simulink model "Ida_FrameWork_Loop"  (R2023a)
settings: Solver=VariableStepAuto  StartTime=0.0  StopTime=inf  RelTol=1e-3
InitFcn:
  | run("Ida_Dynamic.mlx")
undefined symbols (not defined in the file): Cables, Design, init, kappa, n_time_sample, Path, sim_time
libraries: simulink x1
settings Model: PauseTimes=0.01  Creator=Saman  LastModifiedBy=Saman
settings DebuggingCC: UnderSpecifiedDimensionMsg=warning

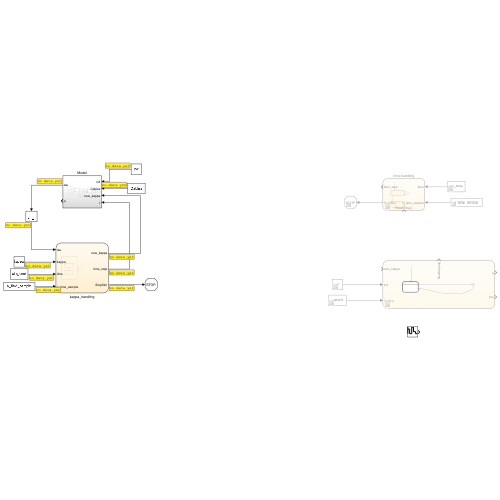
[thumbnail: Simulink's stored preview of the top-level diagram]
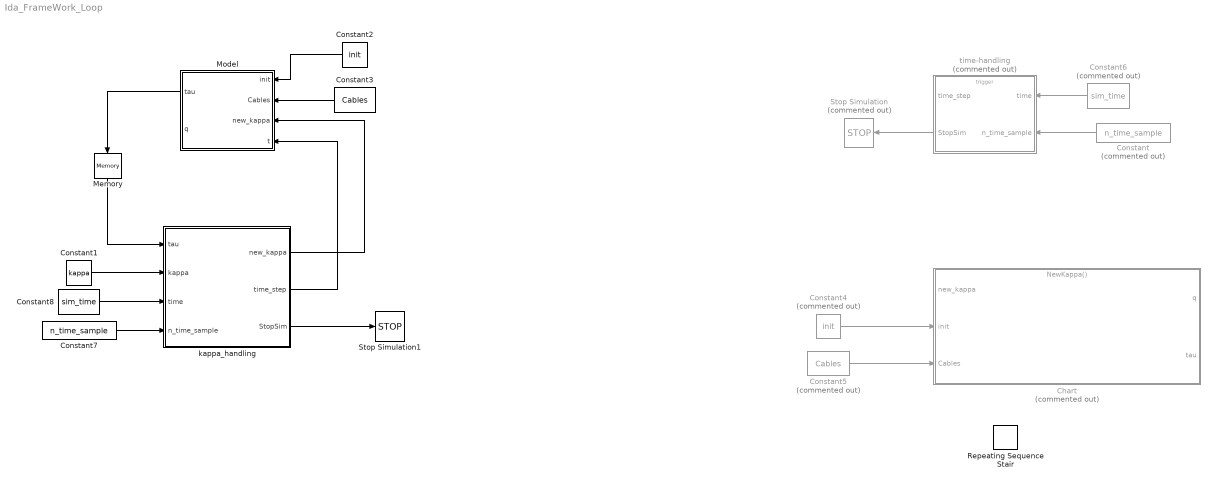
== system Ida_FrameWork_Loop ==
  Chart : Stateflow chart  Commented=on  TreatAsAtomicUnit=on
      settings: PortSchema="{\"entries\":[{\"content\":{\"sides\":[{\"content\":{\"connectorIds\":[\"In1\",\"In2\",\"In3\"]},\"type\":\"ConnectorPlacement.EquallySpacedRectSide\",\"uuid\":\"191c1550-6bd7-40a1-a407-faed922c01f5\"},{\"content\":{\"connectorIds\":[\"Out1\",\"Out2\"],\"side\":\"RIGHT\"},\"type\":\"ConnectorPlacement.EquallySpacedRectSide\",\"uuid\":\"ea9eb825-e49b-447b-9f77-f893937989a1\"},{\"content\":{\"connectorIds\":[\"Out3\"],\"side\":\"TOP\"},\"type\":\"ConnectorPlacement.EquallySpacedRectSide\",\"uuid\":\"63a28030-9dfb-4068-964b-2b00dab3f248\"}]},\"type\":\"ConnectorPlacement.EquallySpacedConnector\",\"uuid\":\"82f8fa03-3b4f-46da-8e57-1f2771fc7109\"}],\"packageUris\":[\"http://schema.mathworks.com/mf0/Connector/R2020b\"],\"version\":\"1.0\"}"
  Constant : Constant  Commented=on  Value=n_time_sample
  Constant1 : Constant  Value=kappa
  Constant2 : Constant  Value=init  OutDataTypeStr=Bus: slBus3
  Constant3 : Constant  Value=Cables  OutDataTypeStr=Bus: slBus1
  Constant4 : Constant  Commented=on  Value=init  OutDataTypeStr=Bus: slBus3
  Constant5 : Constant  Commented=on  Value=Cables  OutDataTypeStr=Bus: slBus1
  Constant6 : Constant  Commented=on  Value=sim_time
  Constant7 : Constant  Value=n_time_sample
  Constant8 : Constant  Value=sim_time
  Memory : Memory
  Model : Subsystem
  Repeating Sequence Stair : simulink/Sources/Repeating Sequence Stair  OutValues=sim_time  tsamp=-1  OutMin=[]  OutMax=[]  OutDataTypeStr=double  OutputDataTypeScalingMode=double  OutDataType=fixdt(0,8)  ConRadixGroup=Best Precision: Vector-wise  OutScaling=2^-12
  Stop Simulation : Stop  Commented=on
  Stop Simulation1 : Stop
  kappa_handling : Stateflow chart  TreatAsAtomicUnit=on
  time-handling : Stateflow chart  Commented=on  TreatAsAtomicUnit=on
  wires:
  Constant4/1 -> Chart/2(init)
  Constant5/1 -> Chart/3(Cables)
  Constant1/1 -> kappa_handling/2(kappa)
  Model/1(tau) -> Memory/1
  Constant3/1 -> Model/2(Cables)
  Constant2/1 -> Model/1(init)
  kappa_handling/1(new_kappa) -> Model/3(new_kappa)
  Memory/1 -> kappa_handling/1(tau)
  Constant6/1 -> time-handling/1(time)
  Constant/1 -> time-handling/2(n_time_sample)
  time-handling/2(StopSim) -> Stop Simulation/1
  kappa_handling/3(StopSim) -> Stop Simulation1/1
  Constant8/1 -> kappa_handling/3(time)
  Constant7/1 -> kappa_handling/4(n_time_sample)
  kappa_handling/2(time_step) -> Model/4(t)

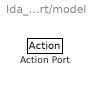
== system Ida_FrameWork_Loop/Chart/model ==
  Action Port : ActionPort
      settings: CopyFcn=Stateflow.SLINSF.SimulinkMan.removeBlockPreDeleteFcn  PreDeleteFcn=Stateflow.SLINSF.SimulinkMan.unsafePredeleteFcn

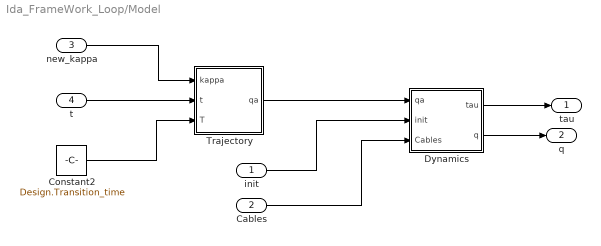
== system Ida_FrameWork_Loop/Model ==
  init : Inport
  Cables : Inport  Port=2
  new_kappa : Inport  Port=3
  t : Inport  Port=4
  Constant2 : Constant  Value=Design.Transition_time
  Dynamics : Subsystem
  Trajectory : Subsystem
  tau : Outport
  q : Outport  Port=2
  wires:
  new_kappa/1 -> Trajectory/1(kappa)
  Dynamics/1(tau) -> tau/1
  Dynamics/2(q) -> q/1
  t/1 -> Trajectory/2(t)
  init/1 -> Dynamics/2(init)
  Cables/1 -> Dynamics/3(Cables)
  Trajectory/1(qa) -> Dynamics/1(qa)
  Constant2/1 -> Trajectory/3(T)

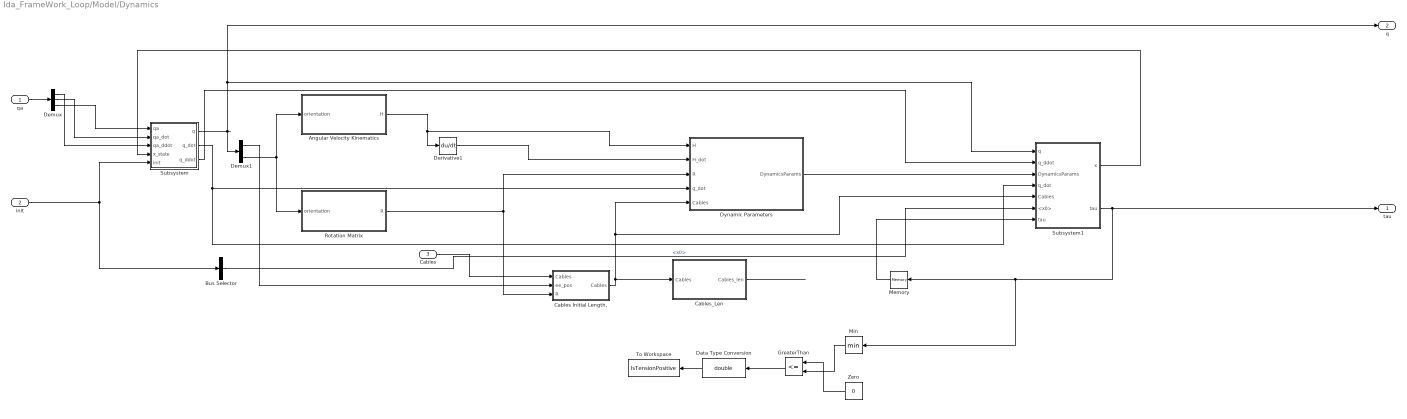
== system Ida_FrameWork_Loop/Model/Dynamics ==
  qa : Inport
  init : Inport  Port=2  OutDataTypeStr=Bus: slBus3
  Cables : Inport  Port=3  OutDataTypeStr=Bus: slBus1
  Angular Velocity Kinematics : MATLAB Function  TreatAsAtomicUnit=on
  Bus Selector : BusSelector  OutputSignals=x0
  Cables Initial Length, : MATLAB Function  TreatAsAtomicUnit=on
  Cables_Len : MATLAB Function  TreatAsAtomicUnit=on
  Data Type Conversion : DataTypeConversion  OutDataTypeStr=double  SaturateOnIntegerOverflow=off  RndMeth=Floor
  Demux : Demux  Outputs=3
  Demux1 : Demux  Outputs=2
  Derivative1 : Derivative
  Dynamic Parameters : MATLAB Function  TreatAsAtomicUnit=on
  GreaterThan : RelationalOperator  Operator=<=  OutDataTypeStr=boolean  RndMeth=Simplest  InputSameDT=off
  Memory : Memory
  Min : MinMax
  Rotation Matrix : MATLAB Function  TreatAsAtomicUnit=on
  Subsystem : Subsystem
  Subsystem1 : Subsystem
  To Workspace : ToWorkspace  VariableName=IsTensionPositive  SaveFormat=Timeseries  SampleTime=-1
  Zero : Constant  Value=0  OutDataTypeStr=Inherit: Inherit via back propagation
  tau : Outport
  q : Outport  Port=2
  wires:
  Cables/1 -> Cables Initial Length,/1("Cables ")
  Angular Velocity Kinematics/1(H) -> Dynamic Parameters/1(H), Derivative1/1
  Derivative1/1 -> Dynamic Parameters/2(H_dot)
  Rotation Matrix/1(R) -> Cables Initial Length,/3(R), Dynamic Parameters/3(R)
  qa/1 -> Demux/1
  init/1 -> Bus Selector/1, Subsystem/5(init)
  Subsystem/1(q) -> q/1, Subsystem1/1(q), Demux1/1
  Demux1/2 -> Rotation Matrix/1(orientation), Angular Velocity Kinematics/1(orientation)
  Demux1/1 -> Cables Initial Length,/2(ee_pos)
  Subsystem/2(q_dot) -> Subsystem1/4(q_dot), Dynamic Parameters/4(q_dot)
  Demux/3 -> Subsystem/1(qa)
  Demux/2 -> Subsystem/2(qa_dot)
  Demux/1 -> Subsystem/3(qa_ddot)
  GreaterThan/1 -> Data Type Conversion/1
  Zero/1 -> GreaterThan/1
  Min/1 -> GreaterThan/2
  Cables Initial Length,/1(Cables) -> Cables_Len/1(Cables), Subsystem1/5(Cables), Dynamic Parameters/5(Cables)
  Cables_Len/1(Cables_len) -> ?
  Data Type Conversion/1 -> To Workspace/1
  Subsystem1/2(tau) -> tau/1, Min/1, Memory/1
  Subsystem/3(q_ddot) -> Subsystem1/2(q_ddot)
  Dynamic Parameters/1(DynamicsParams) -> Subsystem1/3(DynamicsParams)
  Bus Selector/1 -> Subsystem1/6(<x0>)  "<x0>"
  Memory/1 -> Subsystem1/7("tau ")
  Subsystem1/1(x) -> Subsystem/4(x_state)

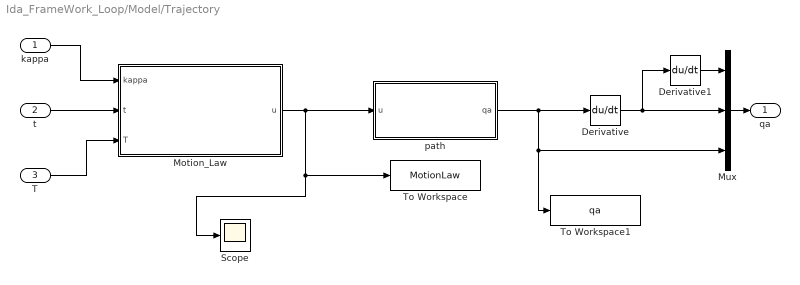
== system Ida_FrameWork_Loop/Model/Trajectory ==
  kappa : Inport
  t : Inport  Port=2
  T : Inport  Port=3
  Derivative : Derivative
  Derivative1 : Derivative
  Motion_Law : MATLAB Function  TreatAsAtomicUnit=on
  Mux : Mux  Inputs=3
  Scope : Scope
  To Workspace : ToWorkspace  VariableName=MotionLaw  SaveFormat=Timeseries  SampleTime=-1
  To Workspace1 : ToWorkspace  VariableName=qa  SaveFormat=Timeseries  SampleTime=-1
  path : MATLAB Function  TreatAsAtomicUnit=on
  qa : Outport
  wires:
  Derivative1/1 -> Mux/1
  Motion_Law/1(u) -> Scope/1, To Workspace/1, path/1(u)
  Derivative/1 -> Derivative1/1, Mux/2
  path/1(qa) -> Derivative/1, To Workspace1/1, Mux/3
  T/1 -> Motion_Law/3(T)
  t/1 -> Motion_Law/2(t)
  Mux/1 -> qa/1
  kappa/1 -> Motion_Law/1(kappa)

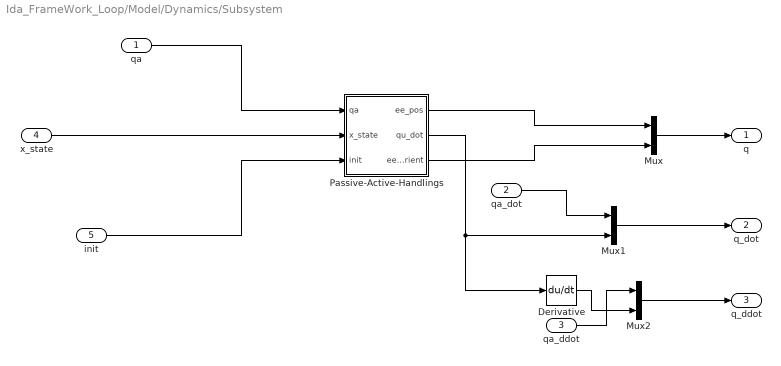
== system Ida_FrameWork_Loop/Model/Dynamics/Subsystem ==
  qa : Inport
  qa_dot : Inport  Port=2
  qa_ddot : Inport  Port=3
  x_state : Inport  Port=4
  init : Inport  Port=5
  Derivative : Derivative
  Mux : Mux  Inputs=2
  Mux1 : Mux  Inputs=2
  Mux2 : Mux  Inputs=2
  Passive-Active-Handlings : Stateflow chart  TreatAsAtomicUnit=on
  q : Outport
  q_dot : Outport  Port=2
  q_ddot : Outport  Port=3
  wires:
  qa/1 -> Passive-Active-Handlings/1(qa)
  Passive-Active-Handlings/3(ee_orient) -> Mux/2
  x_state/1 -> Passive-Active-Handlings/2(x_state)
  init/1 -> Passive-Active-Handlings/3(init)
  Passive-Active-Handlings/1(ee_pos) -> Mux/1
  Mux/1 -> q/1
  qa_dot/1 -> Mux1/1
  Passive-Active-Handlings/2(qu_dot) -> Derivative/1, Mux1/2
  Mux1/1 -> q_dot/1
  Mux2/1 -> q_ddot/1
  qa_ddot/1 -> Mux2/1
  Derivative/1 -> Mux2/2

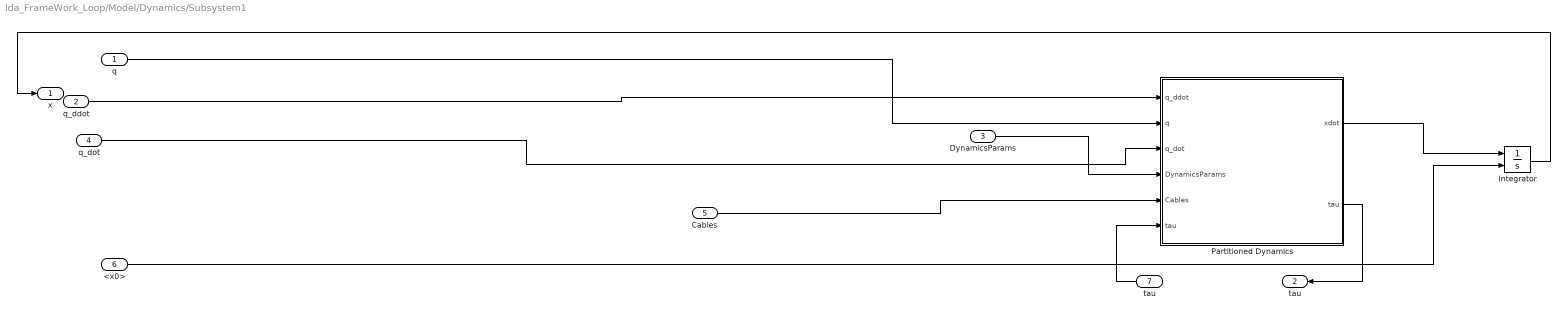
== system Ida_FrameWork_Loop/Model/Dynamics/Subsystem1 ==
  q : Inport
  q_ddot : Inport  Port=2
  DynamicsParams : Inport  Port=3
  q_dot : Inport  Port=4
  Cables : Inport  Port=5
  <x0> : Inport  Port=6
  "tau " : Inport  Port=7
  Integrator : Integrator  InitialConditionSource=external  InitialCondition=init.x0
  Partitioned Dynamics : MATLAB Function  TreatAsAtomicUnit=on
  x : Outport
  tau : Outport  Port=2
  wires:
  Partitioned Dynamics/1(xdot) -> Integrator/1
  q/1 -> Partitioned Dynamics/2(q)
  "tau "/1 -> Partitioned Dynamics/6("tau ")
  <x0>/1 -> Integrator/2
  Partitioned Dynamics/2(tau) -> tau/1
  q_ddot/1 -> Partitioned Dynamics/1(q_ddot)
  DynamicsParams/1 -> Partitioned Dynamics/4(DynamicsParams)
  q_dot/1 -> Partitioned Dynamics/3(q_dot)
  Cables/1 -> Partitioned Dynamics/5(Cables)
  Integrator/1 -> x/1

== matlab function Ida_FrameWork_Loop/Model/Dynamics/Rotation Matrix ==
  data: R output; orientation input
function R = fcn(orientation)
phi=orientation(1);
theta=orientation(2);
chi=orientation(3);

R = [
    cos(theta)*cos(chi),              -cos(theta)*sin(chi),               sin(theta);
    sin(phi)*sin(theta)*cos(chi) + cos(phi)*sin(chi),   -sin(phi)*sin(theta)*sin(chi) + cos(phi)*cos(chi),   -sin(phi)*cos(theta);
    -cos(phi)*sin(theta)*cos(chi) + sin(phi)*sin(chi),  cos(phi)*sin(theta)*sin(chi) + sin(phi)*cos(chi),    cos(phi)*cos(theta)
];

== matlab function Ida_FrameWork_Loop/Model/Dynamics/Angular Velocity Kinematics ==
  data: H output; orientation input size=[3 1]
function H = fcn(orientation)
phi=orientation(1);
theta=orientation(2);
chi=orientation(3);

H =[1 0 sin(theta); 0 cos(phi) -sin(phi)*cos(theta); 0 sin(phi) cos(phi)*cos(theta)];

== matlab function Ida_FrameWork_Loop/Model/Dynamics/Cables Initial Length, ==
  data: Cables input Bus: slBus1; ee_pos input; Cables output; R input; Design parameter Bus: slBus4
function Cables = fcn(Cables,ee_pos, R,Design)

for i=1:Design.Cables_num
    ai=Design.a(:,i);
    di=Design.d(:,i);
    vec = di - ee_pos' - R *ai ;
    Cables(i).Vector=vec';
end

== stateflow chart Ida_FrameWork_Loop/Model/Dynamics/Subsystem/Passive-Active-Handlings ==
  state SoleTransition
    entry,during:
    %q_a(:,i)=qa;
    %q_u(:,i)=qu;
    ee_orient=q_u(1:3);
    ee_pos=qa;
    i=i+1;
  state Store
    entry,during:
    %q_a(:,i)=qa;
    %q_u(:,i)=qu;
    qu=x_state(1:3);
    qu_dot=x_state(4:6);
    ee_orient=qu';
    ee_pos=qa;
    %i=i+1;
  (default) -> (junction 22) : % init
      | {
      | ee_orient=zeros(1,3);
      | ee_pos=zeros(1,3);
      | q_u=init.x0(4:end)';
      | i=1;
      | %q_a=zeros(Design.Cables_num,Design.Transition_time/Design.StepTime);
      | %q_u=zeros(6-Design.Cables_num,Design.Transition_time/Design.StepTime);
      | %x_state=zeros(2*(6-Design.Cables_num),Design.Transition_time/Design.StepTime);
      | %q_u(:,end)=init.x1(3:Design.Cables_num);
      | %x_state(:,1)=init.x0;
      | %x_state(:,end)=init.x1;
      | %q_u(:,end)=init.x1(3:Design.Cables_num);
      | %q_a(:,1)=Path.qa0;
      | %q_a(:,end)=Path.qaT;
      | }
  (junction 22) -> (junction 23) [order 1] : [i==1]
  (junction 23) -> SoleTransition : {
      | %q_u(:,1)=init.x0(3:Design.Cables_num);
      | }
  (junction 22) -> Store [order 2]
  SoleTransition -> Store : [i>1]
  data: Design parameter Bus: slBus4; qa input size=[1 3]; x_state input; Path parameter Bus: slBus2; ee_pos output; qu_dot output; ee_orient output; init input Bus: slBus3; x0 local; q_u local size=[1,3]; i local; qu local

== matlab function Ida_FrameWork_Loop/Model/Dynamics/Cables_Len ==
  data: Cables input Bus: slBus1; Cables_len output
function Cables_len = Cables_Len(Cables)
Cables_len=zeros(numel(Cables),1);
for i=1:numel(Cables)
    Cables_len(i)=norm(Cables(i).Vector);
end

== stateflow chart Ida_FrameWork_Loop/Chart ==
  state model
  (default) -> model : {
      | tau=zeros(3,1);
      | cable_num=3;
      | }
  model -> (junction 16) : [any(tau<0)]
  (junction 16) -> model : {
      |  send(NewKappa)
      | }
  data: sf_internal_action_state_placeholder_data local double size=1 =0; new_kappa input; init input; Cables input; q output; tau output; cable_num local
  events: NewKappa output FUNCTION_CALL_EVENT

== stateflow chart Ida_FrameWork_Loop/kappa_handling ==
  state Positive_Tension_Mode
    state select_time_sample
      du,en:
      time_step=time(index);
      index=index+1;
    state Stop_simulation
      entry:
      send(StopSim);
    (default) -> select_time_sample
    select_time_sample -> Stop_simulation : [index==n_time_sample]
  (default) -> Positive_Tension_Mode : {
      | index=1;
      |  new_kappa=kappa;
      | }
  Positive_Tension_Mode -> Positive_Tension_Mode : [any(tau<0)]{
      | xmin = -100;
      | xmax = 100;
      | new_kappa= xmin + (xmax-xmin)*rand(6,1); % range from -100 to 100
      | }
  data: tau input; kappa input; new_kappa output; xmax local; xmin local; time input; n_time_sample input; time_step output; index local
  events: StopSim output EITHER_EDGE_EVENT; isReset local FUNCTION_CALL_EVENT

== stateflow chart Ida_FrameWork_Loop/time-handling ==
  settings: executeAtInitialization=1
  state select_time_sample
    en,du:
    time_step=time(index);
    index=index+1;
  state Stop_simulation
    entry:
    send(StopSim);
  (default) -> select_time_sample : {index=1}
  select_time_sample -> select_time_sample [order 1] : [ResetTime]
      | {index=1}
  select_time_sample -> Stop_simulation [order 2] : [index==n_time_sample]
  data: time input; time_step output; index local; n_time_sample input
  events: ResetTime input FUNCTION_CALL_EVENT; StopSim output EITHER_EDGE_EVENT

== matlab function Ida_FrameWork_Loop/Model/Trajectory/path ==
  data: u input; qa output; Path parameter Bus: slBus2
function qa = Path(u,Path)

spec=char(Path.spec);
if isequal(spec, 'Line'+0)
    qa=Path.qa0+(Path.qaT-Path.qa0)*u;
else
    error("specify correct Path.spec")

end
end

== matlab function Ida_FrameWork_Loop/Model/Trajectory/Motion_Law ==
  data: kappa input; u output; t input; T input; r parameter
function u = motion_law(kappa, t, T, r)
    
    kappa=kappa';
    
    % Define the degree of the transition polynomial
   

    % Define the coefficients ai using equation (45)
    ai = zeros(1,r+1);
    for i = r+1:2*r+1
        ai(i-r) = (-1)^(i-r-1) * factorial(2*r+1) /((i * factorial(r) * factorial(i-r-1) * factorial(2*r+1-i))) ;
    end

    % Define alpha using equation (53)
    alpha = (1 - sum(kappa .* T.^(2:numel(kappa)+1))) / T;

    % Define gamma as a function of t using equation (53)
    gamma = alpha * t + sum(kappa .* t.^(2:numel(kappa)+1));

    % Calculate u using equation (51)
    u = sum(ai .* gamma.^(r+1:2*r+1));
end

== matlab function Ida_FrameWork_Loop/Model/Dynamics/Subsystem1/Partitioned Dynamics ==
  data: q_ddot input; q input; q_dot input; xdot output; DynamicsParams input Bus: slBus5; Cables input; Design parameter Bus: slBus4; tau output size=[3,1]; tau input size=[3,1]
function [xdot,tau] = fcn(q_ddot, q,q_dot, DynamicsParams,Cables,Design, tau)

%%%%%%%%%%%%%%%%%%%%%%%%%%%%%%%%%%%%% Parametrs Initialization %%%%%%%%%%%%%%%%%%
M=DynamicsParams.M;
C=DynamicsParams.C;
G=DynamicsParams.G;
J=DynamicsParams.J;
Fw=DynamicsParams.Fw;


% Maa=M(1:3,1:3);
% Mau=M(1:3,4:6);
% Mua=M(4:6,1:3);
% Muu=M(4:6,4:6);
%
% Caa=C(1:3,1:3);
% Cau=C(1:3,4:6);
% Cua=C(4:6,1:3);
% Cuu=C(4:6,4:6);


% Define the constants and variables
m = Design.Cables_num; % number of cables
h = 6;% dimension of motion space
n =Design.Cables_num; % number of actuated coordinates
lambda = h - n;% number of unactuated coordinates

% tau = zeros(3,1); % vector of normalized cable tensions

% Compute M, s, B, q, q_dot, q_ddot from the kinematic and dynamic model (not shown here)

% Partition the matrices and vectors according to actuated and unactuated coordinates
% M_aa = M(1:n,1:n);
% M_au = M(1:n,n+1:h);
% M_ua = M(n+1:h,1:n);
% M_uu = M(n+1:h,n+1:h);
% 
% C_aa = C(1:n,1:n);
% C_au = C(1:n,n+1:h);
% C_ua = C(n+1:h,1:n);
% C_uu = C(n+1:h,n+1:h);
% 
% G_a=G(1:n);
% G_u=G(n+1:h);
% 
% B=-J';
% J_a = B(1:n,:);
% J_u = B(n+1:h,:);
% 
% q_a = q(1:n);
% q_u = q(n+1:h);
% 
% q_dot_a = q_dot(1:n);
% q_dot_u = q_dot(n+1:h);
% 
% q_ddot_a = q_ddot(1:n);
% q_ddot_u = q_ddot(n+1:h);

% tau = zeros(3,1);

M_aa = M(1:3,1:3);
M_au = M(1:3,4:6);
M_ua = M(4:6,1:3);
M_uu = M(4:6,4:6);

C_aa = C(1:3,1:3);
C_au = C(1:3,4:6);
C_ua = C(4:6,1:3);
C_uu = C(4:6,4:6);

G_a=G(1:3);
G_u=G(4:6);

B=-J';
J_a = B(1:3,:);
J_u = B(4:6,:);

q_a = q(1:3)';
q_u = q(4:6)';

q_dot_a = q_dot(1:3)';
q_dot_u = q_dot(4:6)';

q_ddot_a = q_ddot(1:3)';
q_ddot_u = q_ddot(4:6)';

% Equation 41: compute the unactuated accelerations as a function of the actuated ones
x=zeros(2*lambda,1);
xdot=zeros(6,1);

x=[q_u;q_dot_u];
q_ddot_u = -M_uu \ (C_ua * q_dot_a + C_uu * q_dot_u + M_ua * q_ddot_a + G_u - J_u * tau);
xdot=[q_dot_u;q_ddot_u];

% Equation 43: compute the vector mu as a function of the actuated accelerations
mu = -C_aa * q_dot_a - C_au * q_dot_u - M_aa * q_ddot_a + M_au * inv (M_uu) * (C_ua * q_dot_a + C_uu * q_dot_u + M_ua * q_ddot_a + G_u) - G_a; % This is the vector of generalized forces for q_a

% Equation 42: compute the normalized cable tensions as a function of the actuated accelerations
tau = inv (M_au * inv (M_uu) * J_u - J_a) * mu;

== matlab function Ida_FrameWork_Loop/Model/Dynamics/Dynamic Parameters ==
  data: DynamicsParams output Bus: slBus5; H input; H_dot input; R input; q_dot input; Cables input Bus: slBus1; Design parameter Bus: slBus4
function DynamicsParams = fcn(H,H_dot,R,q_dot,Cables,Design)



%%%%%%%%%%%%%%%%%%%%%%%%%%%%%%%%%%% Parametrs Initialization %%%%%%%%%%%%%%%%%%
g=Design.g;
Ic=Design.Ic;
Ic=R*Ic*R';
r_p=Design.rho_p;
r_g=R*r_p;
rho_g=[0 -r_g(3) r_g(2); r_g(3) 0 -r_g(1); -r_g(2) r_g(1) 0];
m=Design.m;
omega=q_dot(4:6);
Omega=[0 -omega(3) omega(2); omega(3) 0 -omega(1); -omega(2) omega(1) 0];


Cables_num=Design.Cables_num;
Cables_Length=zeros(Cables_num,1);
Cables_Tension=zeros(Cables_num,1);
Cables_force=zeros(3,Cables_num);

for i = 1:Cables_num
    Cables_Length(i) = norm(Cables(i).Vector);
    Cables_Tension(i)=norm(Cables(i).force)/Cables_Length(i);
    Cables_force(:,i)=Cables(i).force;
end


%%%%%%%%%%%%%%%%%%%%%%%%%%%%%%%%%%%%% Create M_prime matrix %%%%%%%%%%%%%%%%%%  
DynamicsParams.M = [m*eye(3), -m * rho_g * H; 
m * H' * rho_g, H' * Ic * H - m * H' * rho_g^2 * H];
 

%%%%%%%%%%%%%%%%%%%%%%%%%%%%%%%%%%%%% Create C_prime matrix %%%%%%%%%%%%%%%%%%   
DynamicsParams.C = [zeros(3), -m*Omega*rho_g*H + m*rho_g*H_dot;
               zeros(3), H'*((Omega *Ic - m*Omega*rho_g^2)*H +(-rho_g^2 *m +Ic)*H_dot)];

%%%%%%%%%%%%%%%%%%%%%%%%%%%%%%%%%%%%% Create G_prime matrix %%%%%%%%%%%%%%%%%%
fg=m*g;
fc=sum(Cables_force,2);
DynamicsParams.G=[fg;rho_g*fg+rho_g*fc];
% DynamicsParams.G=[fg;rho_g*fg];

%%%%%%%%%%%%%%%%%%%%%%%%%%%%%%%%%%%%% Jacobian matrix %%%%%%%%%%%%%%%%%%

% Preallocate a matrix to hold the row vectors

J = zeros(Cables_num,6);

% Loop over the cables and compute the row vectors
for i = 1:Cables_num
  % Define the variables for the i-th cable
  % rho = Cables(i).Vector/Cables_Length(i); % unit vector along the cable
  rho=Cables(i).Vector;
  
  ap = Design.a(:,i); % attach points vector on platform in body frame

  ag=R*ap; % attach points vector on platform in global frame

  % Compute the skew-symmetric matrix of a
  a_tilde = [0 -ag(3) ag(2); ag(3) 0 -ag(1); -ag(2) ag(1) 0];

  % Compute and assign the row vector of Jq,i
  J(i,:) = [rho,-rho*a_tilde * H];
end

DynamicsParams.J=J(1:3,:);

%%%%%%%%%%%%%%%%%%%%%%%%%%%%%%%%%%%%% Exerted Cables Wrench %%%%%%%%%%%%%%%%%%
DynamicsParams.Fw=-J'*Cables_Tension;
